simulink model "exe_1_3_sim"  (R2022b)
settings: Solver=VariableStepAuto  StartTime=0.0  StopTime=sim_T  RelTol=1e-3
values from neighbouring files (symbols this model uses):
  A = [0, -1/C ... (first row only)    [exe_1_3.m]
  B = [1/C ... (first row only)    [exe_1_3.m]
  C = 1e-3    (= 0.001)    [exe_1_1.m]    (also in exe_1_3.m = [0 R])
  D = [0]    [exe_1_3.m]
settings Model: Creator=nicol  LastModifiedBy=nicol

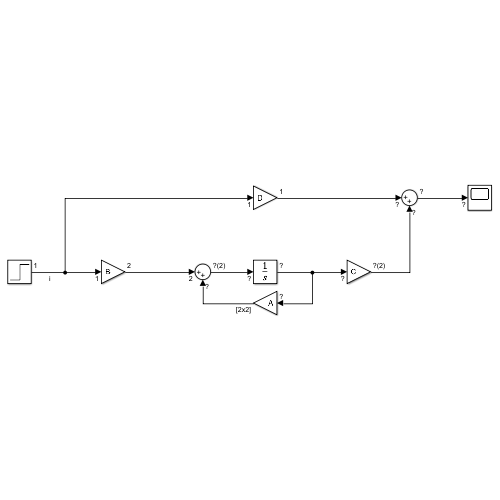
[thumbnail: Simulink's stored preview of the top-level diagram]
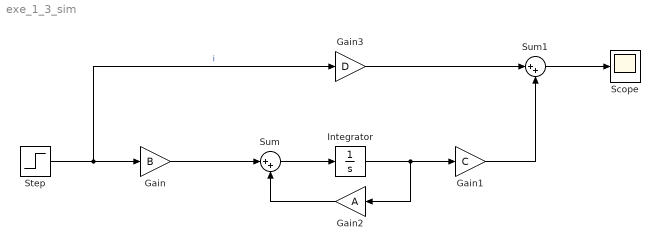
== system exe_1_3_sim ==
  Gain : Gain  Gain=B
  Gain1 : Gain  Gain=C
  Gain2 : Gain  Gain=A
  Gain3 : Gain  Gain=D
  Integrator : Integrator
  Scope : Scope
  Step : Step  Time=0  SampleTime=0
  Sum : Sum  Inputs=|++
  Sum1 : Sum  Inputs=|++
  wires:
  Step/1 -> Gain3/1, Gain/1  "i"
  Gain/1 -> Sum/1
  Sum/1 -> Integrator/1
  Integrator/1 -> Gain2/1, Gain1/1
  Gain2/1 -> Sum/2
  Gain3/1 -> Sum1/1
  Gain1/1 -> Sum1/2
  Sum1/1 -> Scope/1
